simulink model "Shock_Absorber"  (R2018b)
settings: Solver=VariableStepAuto  StartTime=0.0  StopTime=10  RelTol=1e-3
settings Model: Creator=daiba  LastModifiedBy=daiba

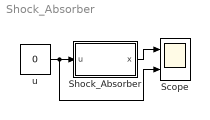
== system Shock_Absorber ==
  Scope : Scope  NumInputPorts=2
  "Shock_Absorber " : Subsystem  mask{m=2, k=0.15, b=0.2, x_zero=0}
      mask prompts: m "Khoi luong vat nang"; k "Do cung lo xo"; b "He so ma sat"; x_zero "Vi tri ban dau"
  u : Constant  Value=0
  wires:
  u/1 -> Scope/2, "Shock_Absorber "/1(u)
  "Shock_Absorber "/1(x) -> Scope/1

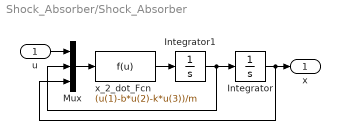
== system Shock_Absorber/Shock_Absorber  ==
  u : Inport
  Integrator : Integrator  InitialCondition=x_zero
  Integrator1 : Integrator
  Mux : Mux  Inputs=3
  x_2_dot_Fcn : Fcn  Expr=(u(1)-b*u(2)-k*u(3))/m
  x : Outport
  wires:
  Mux/1 -> x_2_dot_Fcn/1
  u/1 -> Mux/1
  Integrator/1 -> Mux/3, x/1
  x_2_dot_Fcn/1 -> Integrator1/1
  Integrator1/1 -> Mux/2, Integrator/1
